simulink library "auxvars_lib"  (Simulink 7.2)
settings: Solver=ode45  SolverMode=SingleTasking  StartTime=0.0  StopTime=10.0  RelTol=1e-3
libraries: Euler_to_DCM_lib x1, Vb_Converter_lib x1, simulink x1
settings Model: Creator=amurch  LastModifiedBy=mahill  ExtModeAutoUpdateStatusClock=off

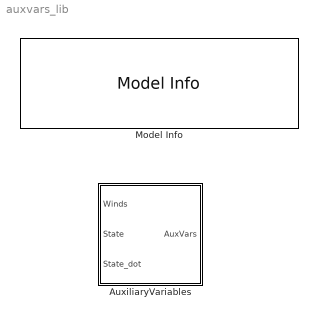
== system auxvars_lib ==
  AuxiliaryVariables : Subsystem
  Model Info : simulink/Model-Wide Utilities/Model Info  SystemSampleTime=-1  InitialBlockCM=None  BlockCM=None  Frame=on  DisplayStringWithTags=|  HorizontalTextAlignment=Center  LeftAlignmentValue=0.5  SourceBlockDiagram=auxvars_lib  TagMaxNumber=20
      | Auxiliary Variables Library
      | %<ModelVersion>
      | Las modified by %<LastModifiedBy> on %<LastModificationDate>

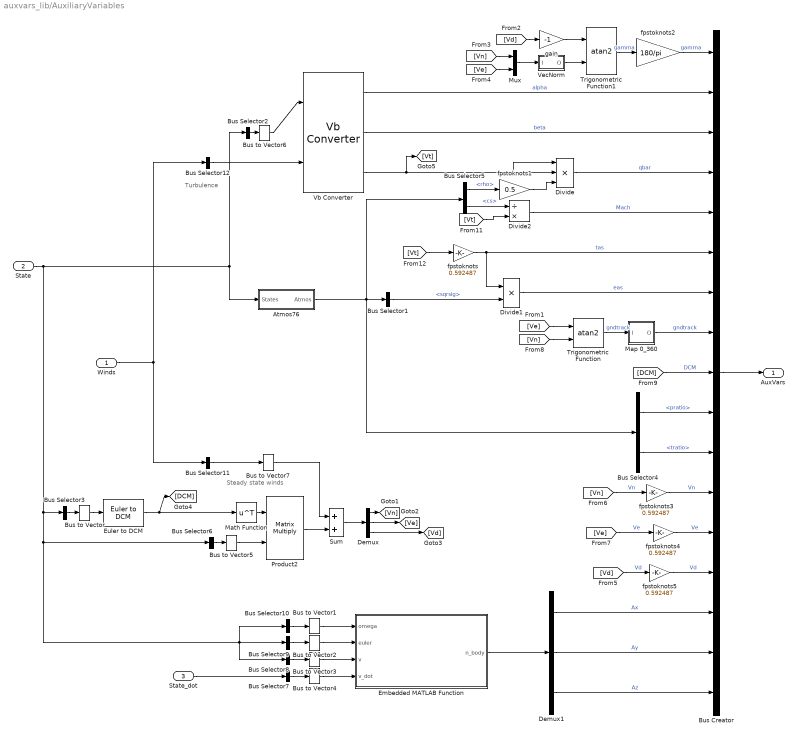
== system auxvars_lib/AuxiliaryVariables ==
  note: Steady state winds
  note: Turbulence
  Winds : Inport  PortDimensions=6  OutDataType=sfix(16)  OutScaling=2^0
  State : Inport  Port=2  OutDataType=sfix(16)  OutScaling=2^0
  State_dot : Inport  Port=3  OutDataType=sfix(16)  OutScaling=2^0
  Atmos76 : Subsystem
  Bus Creator : BusCreator  Inputs=17
  Bus Selector1 : BusSelector  OutputSignals=sqrsig
  Bus Selector10 : BusSelector  OutputSignals=pb,qb,rb  OutputAsBus=on
  Bus Selector11 : BusSelector  OutputSignals=NorthWind,EastWind,VerticalWind  OutputAsBus=on
  Bus Selector12 : BusSelector  OutputSignals=turb_u_body,turb_v_body,turb_w_body  OutputAsBus=on
  Bus Selector2 : BusSelector  OutputSignals=ub,vb,wb  OutputAsBus=on
  Bus Selector3 : BusSelector  OutputSignals=phi,theta,psi  OutputAsBus=on
  Bus Selector4 : BusSelector  OutputSignals=pratio,tratio
  Bus Selector5 : BusSelector  OutputSignals=rho,cs
  Bus Selector6 : BusSelector  OutputSignals=ub,vb,wb  OutputAsBus=on
  Bus Selector7 : BusSelector  OutputSignals=ub_dot,vb_dot,wb_dot  OutputAsBus=on
  Bus Selector8 : BusSelector  OutputSignals=ub,vb,wb  OutputAsBus=on
  Bus Selector9 : BusSelector  OutputSignals=phi,theta,psi  OutputAsBus=on
  Bus to Vector{,1..7} (8 alike) : BusToVector
  Demux : Demux  Outputs=3
  Demux1 : Demux  Outputs=3
  Divide : Product  Inputs=***  OutDataType=sfix(16)  OutScaling=2^-10
  Divide1 : Product  OutDataType=sfix(16)  OutScaling=2^-10
  Divide2 : Product  Inputs=/*  OutDataType=sfix(16)  OutScaling=2^-10
  Embedded MATLAB Function : Stateflow chart
  Euler to DCM : Euler_to_DCM_lib/Euler to DCM  SystemSampleTime=-1
  Map 0_360 : Subsystem
  Math Function : Math  Operator=transpose  OutDataType=sfix(16)  OutScaling=2^0  SaturateOnIntegerOverflow=on
  Mux : Mux  Inputs=2
  Product2 : Product  Multiplication=Matrix(*)  OutDataType=sfix(16)  OutScaling=2^0  RndMeth=Zero
  Sum : Sum  OutDataType=sfix(16)  OutScaling=2^0
  Trigonometric Function : Trigonometry  Operator=atan2
  Trigonometric Function1 : Trigonometry  Operator=atan2
  Vb Converter : Vb_Converter_lib/Vb Converter  SystemSampleTime=-1
  VecNorm : Subsystem
  fpstoknots{,3..5} (4 alike) : Gain  Gain=0.592487  ParameterDataType=sfix(16)  ParameterScaling=2^0  OutDataType=sfix(16)  OutScaling=2^0
  fpstoknots1 : Gain  Gain=0.5  ParameterDataType=sfix(16)  ParameterScaling=2^0  OutDataType=sfix(16)  OutScaling=2^0
  fpstoknots2 : Gain  Gain=180/pi  ParameterDataType=sfix(16)  ParameterScaling=2^0  OutDataType=sfix(16)  OutScaling=2^0
  gain : Gain  Gain=-1  ParameterDataType=sfix(16)  ParameterScaling=2^0  OutDataType=sfix(16)  OutScaling=2^0
  AuxVars : Outport  OutDataType=sfix(16)  OutScaling=2^0
  wires:
  fpstoknots2/1 -> Bus Creator/1  "gamma"
  VecNorm/1(O) -> Trigonometric Function1/2
  [Ve] -> Mux/2
  [Vn] -> Mux/1
  Mux/1 -> VecNorm/1(I)
  [Vd] -> gain/1
  gain/1 -> Trigonometric Function1/1
  Trigonometric Function1/1 -> fpstoknots2/1  "gamma"
  Demux/3 -> [Vd]
  Euler to DCM/1 -> [DCM], Math Function/1
  Divide/1 -> Bus Creator/4  "qbar"
  fpstoknots1/1 -> Divide/3
  Bus Selector5/1 -> fpstoknots1/1  "<rho>"
  Vb Converter/2 -> Bus Creator/3  "beta"
  Vb Converter/1 -> Bus Creator/2  "alpha"
  Bus Selector1/1 -> Divide1/2  "<sqrsig>"
  Vb Converter/3 -> Divide/2, Divide/1, [Vt]
  Winds/1 -> Bus Selector11/1, Bus Selector12/1
  fpstoknots/1 -> Divide1/1, Bus Creator/6  "tas"
  Atmos76/1(Atmos) -> Bus Selector5/1, Bus Selector1/1, Bus Selector4/1
  State/1 -> Bus Selector2/1, Atmos76/1(States), Bus Selector9/1, Bus Selector10/1, Bus Selector8/1, Bus Selector6/1, Bus Selector3/1
  Divide1/1 -> Bus Creator/7  "eas"
  [Ve] -> fpstoknots4/1  "Ve"
  [Vn] -> fpstoknots3/1  "Vn"
  [Vd] -> fpstoknots5/1  "Vd"
  Bus Selector4/1 -> Bus Creator/10  "<pratio>"
  Bus Selector4/2 -> Bus Creator/11  "<tratio>"
  [Ve] -> Trigonometric Function/1
  [Vn] -> Trigonometric Function/2
  Map 0_360/1(O) -> Bus Creator/8  "gndtrack"
  Trigonometric Function/1 -> Map 0_360/1(I)  "gndtrack"
  Bus Selector5/2 -> Divide2/1  "<cs>"
  Divide2/1 -> Bus Creator/5  "Mach"
  fpstoknots3/1 -> Bus Creator/12  "Vn"
  fpstoknots4/1 -> Bus Creator/13  "Ve"
  fpstoknots5/1 -> Bus Creator/14  "Vd"
  [DCM] -> Bus Creator/9  "DCM"
  [Vt] -> Divide2/2
  [Vt] -> fpstoknots/1
  Bus Creator/1 -> AuxVars/1
  Bus Selector7/1 -> Bus to Vector4/1
  State_dot/1 -> Bus Selector7/1
  Bus Selector8/1 -> Bus to Vector3/1
  Bus Selector9/1 -> Bus to Vector2/1
  Bus Selector10/1 -> Bus to Vector1/1
  Demux1/1 -> Bus Creator/15  "Ax"
  Demux1/2 -> Bus Creator/16  "Ay"
  Demux1/3 -> Bus Creator/17  "Az"
  Embedded MATLAB Function/1(n_body) -> Demux1/1
  Demux/2 -> [Ve]
  Demux/1 -> [Vn]
  Math Function/1 -> Product2/1
  Bus Selector6/1 -> Bus to Vector5/1
  Bus Selector3/1 -> Bus to Vector/1
  Bus to Vector/1 -> Euler to DCM/1
  Bus to Vector1/1 -> Embedded MATLAB Function/1(omega)
  Bus to Vector2/1 -> Embedded MATLAB Function/2(euler)
  Bus to Vector3/1 -> Embedded MATLAB Function/3(v)
  Bus to Vector4/1 -> Embedded MATLAB Function/4(v_dot)
  Bus to Vector5/1 -> Product2/2
  Bus Selector2/1 -> Bus to Vector6/1
  Bus to Vector6/1 -> Vb Converter/1
  Bus to Vector7/1 -> Sum/1
  Product2/1 -> Sum/2
  Sum/1 -> Demux/1
  Bus Selector11/1 -> Bus to Vector7/1
  Bus Selector12/1 -> Vb Converter/2

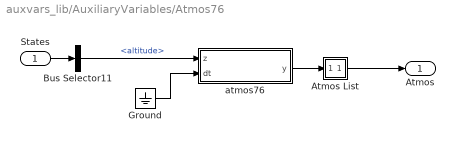
== system auxvars_lib/AuxiliaryVariables/Atmos76 ==
  States : Inport  OutDataType=sfix(16)  OutScaling=2^0
  Atmos List : Subsystem
  Bus Selector11 : BusSelector  OutputSignals=altitude
  Ground : Ground
  atmos76 : Stateflow chart
  Atmos : Outport  OutDataType=sfix(16)  OutScaling=2^0
  wires:
  atmos76/1(y) -> Atmos List/1(I)
  Bus Selector11/1 -> atmos76/1(z)  "<altitude>"
  States/1 -> Bus Selector11/1
  Atmos List/1(O) -> Atmos/1
  Ground/1 -> atmos76/2(dt)

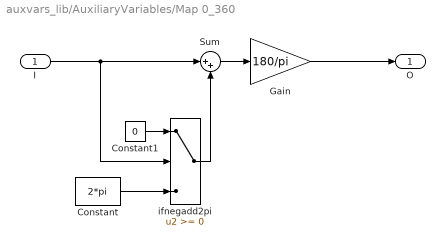
== system auxvars_lib/AuxiliaryVariables/Map 0_360 ==
  I : Inport  OutDataType=sfix(16)  OutScaling=2^0
  Constant : Constant  Value=2*pi  OutDataType=sfix(16)  OutScaling=2^0
  Constant1 : Constant  Value=0  OutDataType=sfix(16)  OutScaling=2^0
  Gain : Gain  Gain=180/pi  ParameterDataType=sfix(16)  ParameterScaling=2^0  OutDataType=sfix(16)  OutScaling=2^0
  Sum : Sum  Inputs=|++  OutDataType=sfix(16)  OutScaling=2^0
  ifnegadd2pi : Switch
  O : Outport  OutDataType=sfix(16)  OutScaling=2^0
  wires:
  I/1 -> Sum/1, ifnegadd2pi/2
  Sum/1 -> Gain/1
  ifnegadd2pi/1 -> Sum/2
  Constant/1 -> ifnegadd2pi/3
  Constant1/1 -> ifnegadd2pi/1
  Gain/1 -> O/1

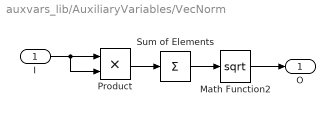
== system auxvars_lib/AuxiliaryVariables/VecNorm ==
  I : Inport  OutDataType=sfix(16)  OutScaling=2^0
  Math Function2 : Math  Operator=sqrt  OutDataType=sfix(16)  OutScaling=2^0  SaturateOnIntegerOverflow=on
  Product : Product  OutDataType=sfix(16)  OutScaling=2^0  RndMeth=Zero
  Sum of Elements : Sum  Inputs=+  OutDataType=sfix(16)  OutScaling=2^-10
  O : Outport  OutDataType=sfix(16)  OutScaling=2^0
  wires:
  Sum of Elements/1 -> Math Function2/1
  Product/1 -> Sum of Elements/1
  I/1 -> Product/2, Product/1
  Math Function2/1 -> O/1

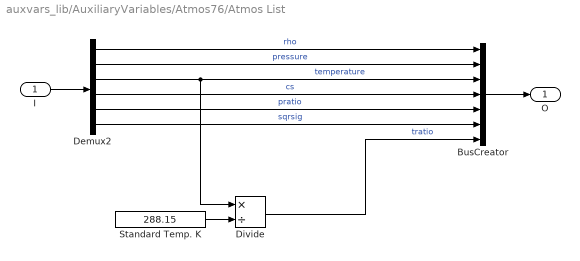
== system auxvars_lib/AuxiliaryVariables/Atmos76/Atmos List ==
  I : Inport  OutDataType=sfix(16)  OutScaling=2^0
  BusCreator : BusCreator  Inputs=7
  Demux2 : Demux  Outputs=6
  Divide : Product  Inputs=*/  OutDataType=sfix(16)  OutScaling=2^-10
  Standard Temp. K : Constant  Value=288.15  OutDataType=sfix(16)  OutScaling=2^0
  O : Outport  OutDataType=sfix(16)  OutScaling=2^0
  wires:
  Demux2/6 -> BusCreator/6  "sqrsig"
  Demux2/5 -> BusCreator/5  "pratio"
  Demux2/4 -> BusCreator/4  "cs"
  Demux2/3 -> BusCreator/3, Divide/1  "temperature"
  Demux2/2 -> BusCreator/2  "pressure"
  Demux2/1 -> BusCreator/1  "rho"
  I/1 -> Demux2/1
  BusCreator/1 -> O/1
  Standard Temp. K/1 -> Divide/2
  Divide/1 -> BusCreator/7  "tratio"

== matlab function AuxiliaryVariables/Atmos76/atmos76 ==
  data: z input double; y output double; dt input double
function y = layer1atm(z,dt)
% Author: Kevin Cunningham          April 20, 1992    
% Modified: Dave Cox                Aug, 14, 2008

y=zeros(6,1);

%dt=0;  % Standard Temp forced.

%    --- constants from 1976 std. atmosphere
r     = 1716.55915670803;
gamma = 1.4;
g     = 32.17405;
re    = 20855531.5;
tsl   = 288.15 * 1.8;
psl   = 2116.22;
hsl   = 0.;
sldens = 0.0023769;                 % atmospheric density at sea level
slpr   = 2116.220;                  % sea level pressure, psf

%---------------------------------------------------------------------
%    conversion from metric lapse rate to english lapse rate
%    meters/0.3048 = ft
%    Kelvin * 1.8 = Rankine
rm2ft = 1000.0/0.3048;
conlapse = 1.8/rm2ft;

%  ---- convert geometric alt. to geopotential alt.
h     = (re*z)/(re+z);
 
%  ---- ensure we are in layer one (based on geopotential alt)
if (h > 11*rm2ft) % 11 km
  %fprintf(1,'Error, atmosphere model out of range %f, Limiting...\n',h);
  h=11*rm2ft;
end
if (h<0)
  %fprintf(1,'Error, atmosphere model out of range %f, Limiting...\n',h);
  h=0;
end

a1     = -6.5*conlapse;
t1     = tsl + a1*(h-hsl);
del1   = (t1/tsl)^(-g/r/a1);
p1     = del1 * psl;

%   ---- apply temperature increment from standard day*/
t1     = t1 + dt;

%   ---- calculate density from eqn. of state w/ corrected temp.*/
rho1   = p1 / (r * t1);
 
%   ---- calculate speed of sound w/ corrected temp.*/
c1     = sqrt(gamma * (r * t1));
 

% Calculate outputs
y(1) = rho1;
y(2) = p1;
y(3) = t1 / 1.8; % output temperature  in Kelvin
y(4) = c1;
y(5) = y(2) / slpr;         % pressure ratio
y(6) = sqrt(y(1)/sldens);   % SQUARE ROOT OF DENSITY RATIO

== matlab function AuxiliaryVariables/Embedded MATLAB Function ==
  data: omega input double; euler input double; v input double; n_body output double; v_dot input double
function n_body = accels(omega,euler,v,v_dot)
% Compute body-axis accelerometer measurements.  
% Inputs:
%       omega: body-axis angular rates, [p q r], in rad/sec
%       euler: Euler angles, [phi theta psi], in rad
%           v: body-axis velocities, [u v w], ft/sec
%       v_dot: body-axis accelerations, [udot vdot wdot], ft/sec^2
%
%
% Author: Austin Murch (Austin.M.Murch@nasa.gov)
% Created: 2/19/2008

g0    = 32.174;
phi   = euler(1);
theta = euler(2);

n_body = (v_dot + cross(omega,v))/g0 - [-sin(theta); cos(theta)*sin(phi); cos(theta)*cos(phi)];
